simulink model "practica1"  (R2024b)
settings: Solver=VariableStepAuto  StartTime=0.0  StopTime=5  RelTol=1e-3
InitFcn:
  | ip = 0.0079;
  | Mc = 0.7031;
  | Lp = 0.3302;
  | Mp = 0.23;
  | Fc = 0;
  | Beq = 4.3;
  | g = 9.81;
  | Bp = 0.0024;
settings Model: LastModifiedBy=52332

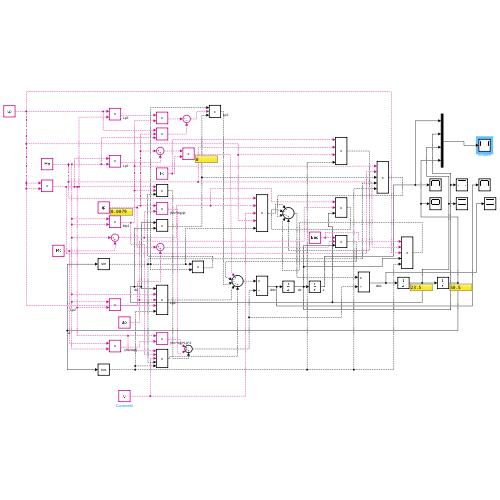
[thumbnail: Simulink's stored preview of the top-level diagram]
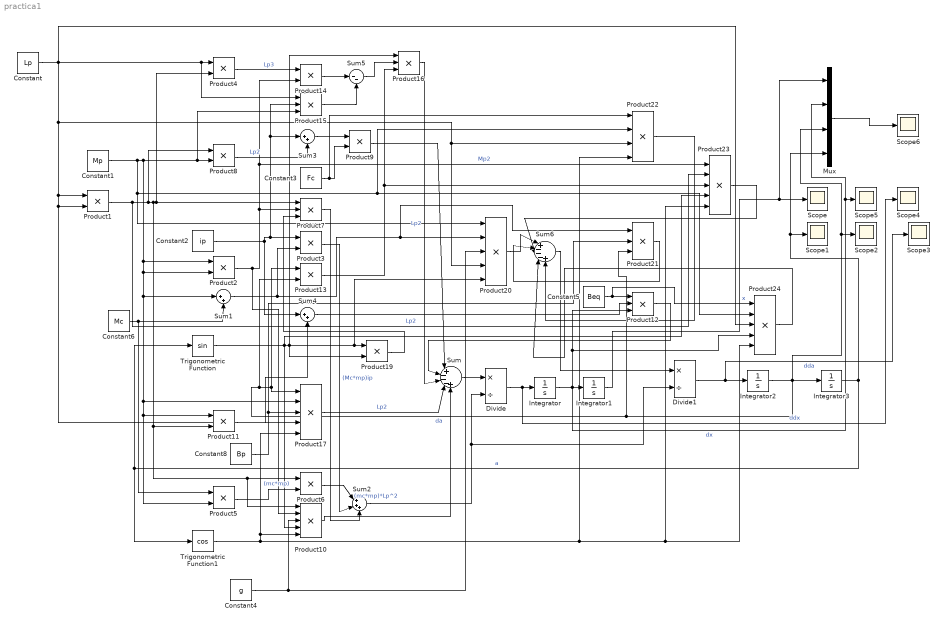
== system practica1 ==
  Constant : Constant  Value=Lp
  Constant1 : Constant  Value=Mp
  Constant2 : Constant  Value=ip
  Constant3 : Constant  Value=Fc
  Constant4 : Constant  Value=g
  Constant5 : Constant  Value=Beq
  Constant6 : Constant  Value=Mc
  Constant8 : Constant  Value=Bp
  Divide : Product  Inputs=*/
  Divide1 : Product  Inputs=*/
  Integrator : Integrator
  Integrator1 : Integrator
  Integrator2 : Integrator
  Integrator3 : Integrator  InitialCondition=pi/180
  Mux : Mux
  Product{1..6,8..9,11,13..14,19} (12 alike) : Product
  Product{10,17,20,23..24} (5 alike) : Product  Inputs=5
  Product{7,12,15..16,21} (5 alike) : Product  Inputs=3
  Product22 : Product  Inputs=4
  Scope{,1..6} (7 alike) : Scope
      Scope settings: Tag=x  Description=x
      Scope1 settings: Tag=a  Description=a
      Scope2 settings: Tag=a  Description=a
      Scope3 settings: Tag=a  Description=a
      Scope4 settings: Tag=x  Description=x
      Scope5 settings: Tag=x  Description=x
      Scope6 settings: Tag=a  Description=a
  Sum : Sum  Inputs=|+---+
  Sum1 : Sum  Inputs=|++
  Sum2 : Sum  Inputs=|+++
  Sum3 : Sum  Inputs=|++
  Sum4 : Sum  Inputs=|++
  Sum5 : Sum  Inputs=|--
  Sum6 : Sum  Inputs=|+---+
  Trigonometric Function : Trigonometry
  Trigonometric Function1 : Trigonometry  Operator=cos
  wires:
  Product12/1 -> Sum/2
  Integrator1/1 -> Mux/1, Scope/1  "x"
  Sum/1 -> Divide/1
  Product16/1 -> Sum/3  "Lp2"
  Sum2/1 -> Divide1/2, Divide/2
  Product9/1 -> Sum/1
  Constant8/1 -> Product21/2, Product17/3
  Integrator2/1 -> Product13/1, Product17/1, Product13/2, Product21/3, Integrator3/1, Mux/3, Scope2/1  "da"
  Sum1/1 -> Product21/1, Product20/2, Product3/2
  Product6/1 -> Sum2/1  "(mc*mp)*Lp^2"
  Product8/1 -> Sum3/2  "Lp2"
  Product4/1 -> Product14/1  "Lp3"
  Trigonometric Function/1 -> Product10/4, Product20/5, Product19/1, Product19/2, Product16/1, Product23/4
  Constant1/1 -> Product22/2, Product24/2, Product20/1, Product5/2, Product11/1, Product17/2, Sum1/1, Product2/2, Product2/1, Product8/2, Product15/3
  Trigonometric Function1/1 -> Product17/5, Product10/5, Product24/5, Product23/5, Product22/4
  Product14/1 -> Sum5/1
  Product2/1 -> Product10/2, Product23/1, Product14/2, Product7/2  "Mp2"
  Integrator/1 -> Mux/2, Scope5/1, Product12/3, Product24/4, Integrator1/1  "dx"
  Sum4/1 -> Product12/2
  Product1/1 -> Product23/2, Product10/1, Product6/1, Product11/2, Product4/2, Product7/1, Product8/1  "Lp2"
  Product17/1 -> Sum/4  "Lp2"
  Constant2/1 -> Product15/2, Sum3/1, Product3/1, Sum4/1
  Integrator3/1 -> Trigonometric Function1/1, Trigonometric Function/1, Mux/4, Scope1/1  "a"
  Constant6/1 -> Product5/1, Sum1/2
  Constant5/1 -> Product24/1, Product12/1
  Constant/1 -> Product22/3, Product20/4, Product17/4, Product1/2, Product1/1, Product15/1, Product4/1, Product24/3
  Product5/1 -> Product6/2  "(mc*mp)"
  Constant4/1 -> Product20/3, Product10/3
  Sum3/1 -> Product9/1
  Product11/1 -> Sum4/2
  Constant3/1 -> Product22/1, Product9/2
  Product7/1 -> Sum2/3
  Product3/1 -> Sum2/2  "(Mc*mp)ip"
  Sum5/1 -> Product16/2
  Product13/1 -> Product23/3, Product16/3
  Divide/1 -> Scope4/1, Integrator/1  "ddx"
  Product15/1 -> Sum5/2
  Product10/1 -> Sum/5
  Divide1/1 -> Scope3/1, Integrator2/1  "dda"
  Product19/1 -> Product7/3
  Product20/1 -> Sum6/1
  Product21/1 -> Sum6/2
  Product22/1 -> Sum6/5
  Product23/1 -> Sum6/3
  Product24/1 -> Sum6/4
  Sum6/1 -> Divide1/1
  Mux/1 -> Scope6/1
